simulink model "gyak3"  (R2018a)
settings: Solver=VariableStepAuto  StartTime=0.0  StopTime=100  RelTol=1e-3
values from neighbouring files (symbols this model uses):
  A = [0 1 0; 0 0 omega^2; 0 1 -1/tao]    [Repcsi.m]    (also in lefekezes_2d.m = [0 1 0 0;0 -mu/M 0 0;0 0 0 1;0 0 0 -mu/M]; test_lefekezes.m = [0 1; 0 -mu/M])
  A_zart = A-B*K    [Repcsi.m]    (also in lefekezes_2d.m; test_lefekezes.m)
  B = [0; omega^2; 0]    [Repcsi.m]    (also in lefekezes_2d.m = [0 0;1/M 0;0 0;0 1/M]; test_lefekezes.m = [0; 1/M])
  B_zart = zeros(size(B))    [Repcsi.m]    (also in lefekezes_2d.m; test_lefekezes.m)
  C = [1 0 0]    [Repcsi.m]    (also in lefekezes_2d.m = [1 0 0 0;0 0 1 0]; test_lefekezes.m = [1 0])
  K = inv(R)*B'*P    [Repcsi.m]    (also in lefekezes_2d.m; test_lefekezes.m)
  x0 = [20; 2; 7]    [Repcsi.m]    (also in lefekezes_2d.m = [100; 10; 30; 70]; test_lefekezes.m = [10; 10])
settings Model: Creator=alfac  LastModifiedBy=alfac

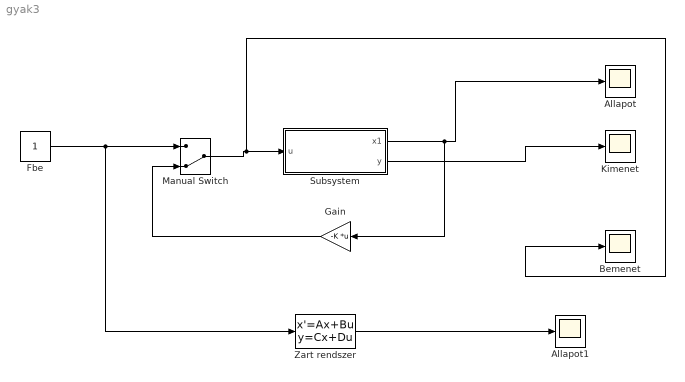
== system gyak3 ==
  Allapot : Scope
  Allapot1 : Scope
  Bemenet : Scope
  Fbe : Constant
  Gain : Gain  Gain=-K  Multiplication=Matrix(K*u)
  Kimenet : Scope
  Manual Switch : ManualSwitch  CurrentSetting=0
  Subsystem : Subsystem
  Zart rendszer : StateSpace  A=A_zart  B=B_zart  C=eye(2)  D=[0;0]  InitialCondition=x0
  wires:
  Gain/1 -> Manual Switch/2
  Fbe/1 -> Manual Switch/1, Zart rendszer/1
  Subsystem/1(x1) -> Allapot/1, Gain/1
  Manual Switch/1 -> Bemenet/1, Subsystem/1(u)
  Subsystem/2(y) -> Kimenet/1
  Zart rendszer/1 -> Allapot1/1

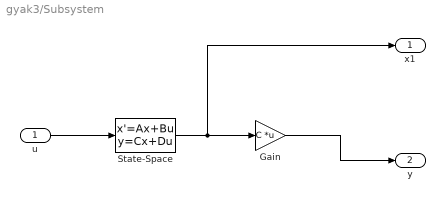
== system gyak3/Subsystem ==
  u : Inport
  Gain : Gain  Gain=C  Multiplication=Matrix(K*u)
  State-Space : StateSpace  A=A  B=B  C=eye(2)  D=[0; 0]  InitialCondition=x0
  x1 : Outport
  y : Outport  Port=2
  wires:
  State-Space/1 -> x1/1, Gain/1
  u/1 -> State-Space/1
  Gain/1 -> y/1
